simulink model "optimized_airport_sim_2"  (R2021a)
settings: Solver=VariableStepAuto  StartTime=0.0  StopTime=1e5  RelTol=1e-3
undefined symbols (not defined in the file): m, n
(part 1 of 2)
settings Model: Creator=hagarusama  LastModifiedBy=hagarusama

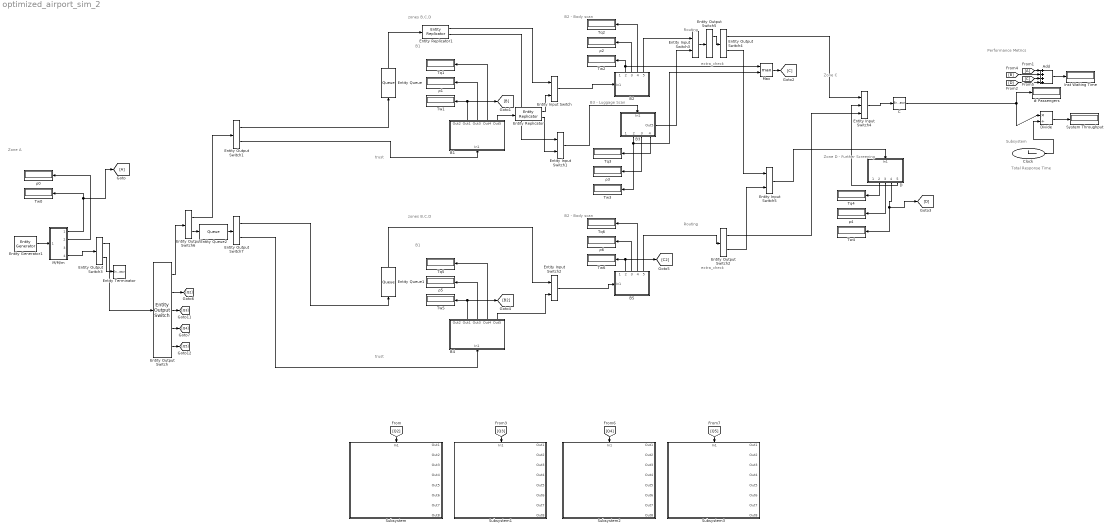
== system optimized_airport_sim_2 ==
  note: B1
  note: zones B,C,D
  note: Zone C
  note: B3 -
      | Luggage
      | Scan
  note: Subsystem
  note: Routing
  note: Zone D -
      |
      | Further
      | Screening
  note: Total Response Time
  note: B2 -
      | Body
      | scan
  note: Performance Metrics
  note: trust
  note: Zone A
  note: extra_check
  note: B1
  note: zones B,C,D
  note: Routing
  note: B2 -
      | Body
      | scan
  note: trust
  note: extra_check
  # Passengers : Display
  Add : Sum  Inputs=++++  SaturateOnIntegerOverflow=on
  B1 : Subsystem
  B2 : Subsystem
      settings: PortSchema="{\"entries\":[{\"content\":{\"sides\":[{\"content\":{\"connectorIds\":[]},\"type\":\"ConnectorPlacement.EquallySpacedRectSide\",\"uuid\":\"7ea955c4-59a0-4b16-a665-3c7419b36f79\"},{\"content\":{\"connectorIds\":[\"Out1\",\"Out2\",\"Out3\",\"Out4\",\"Out5\"],\"side\":\"RIGHT\"},\"type\":\"ConnectorPlacement.EquallySpacedRectSide\",\"uuid\":\"a8a3c229-e196-4360-bdfa-8ef645b2ce9c\"},{\"content\":{\"connectorIds\":[\"In1\"],\"side\":\"TOP\"},\"type\":\"ConnectorPlacement.EquallySpacedRectSide\",\"uuid\":\"5260f7b5-f6e8-463a-b0c5-598c56357d98\"}]},\"type\":\"ConnectorPlacement.EquallySpacedConnector\",\"uuid\":\"58c66fb9-1797-41d8-b8ed-62a065428871\"}],\"packageUris\":[\"http://schema.mathworks.com/mf0/Connector/R2020b\"],\"version\":\"1.0\"}"
  B3 : Subsystem
      settings: PortSchema="{\"entries\":[{\"content\":{\"sides\":[{\"content\":{\"connectorIds\":[\"In1\"]},\"type\":\"ConnectorPlacement.EquallySpacedRectSide\",\"uuid\":\"7ea955c4-59a0-4b16-a665-3c7419b36f79\"},{\"content\":{\"connectorIds\":[\"Out1\",\"Out2\",\"Out3\",\"Out4\"],\"side\":\"RIGHT\"},\"type\":\"ConnectorPlacement.EquallySpacedRectSide\",\"uuid\":\"a8a3c229-e196-4360-bdfa-8ef645b2ce9c\"},{\"content\":{\"connectorIds\":[],\"side\":\"TOP\"},\"type\":\"ConnectorPlacement.EquallySpacedRectSide\",\"uuid\":\"5260f7b5-f6e8-463a-b0c5-598c56357d98\"},{\"content\":{\"connectorIds\":[\"Out5\"],\"side\":\"BOTTOM\"},\"type\":\"ConnectorPlacement.EquallySpacedRectSide\",\"uuid\":\"b778f381-c9da-4203-8e39-7c353a561693\"}]},\"type\":\"ConnectorPlacement.EquallySpacedConnector\",\"uuid\":\"58c66fb9-1797-41d8-b8ed-62a065428871\"}],\"packageUris\":[\"http://schema.mathworks.com/mf0/Connector/R2020b\"],\"version\":\"1.0\"}"
  B4 : Subsystem
  B5 : Subsystem
      settings: PortSchema="{\"entries\":[{\"content\":{\"sides\":[{\"content\":{\"connectorIds\":[]},\"type\":\"ConnectorPlacement.EquallySpacedRectSide\",\"uuid\":\"7ea955c4-59a0-4b16-a665-3c7419b36f79\"},{\"content\":{\"connectorIds\":[\"Out1\",\"Out2\",\"Out3\",\"Out4\",\"Out5\"],\"side\":\"RIGHT\"},\"type\":\"ConnectorPlacement.EquallySpacedRectSide\",\"uuid\":\"a8a3c229-e196-4360-bdfa-8ef645b2ce9c\"},{\"content\":{\"connectorIds\":[\"In1\"],\"side\":\"TOP\"},\"type\":\"ConnectorPlacement.EquallySpacedRectSide\",\"uuid\":\"5260f7b5-f6e8-463a-b0c5-598c56357d98\"}]},\"type\":\"ConnectorPlacement.EquallySpacedConnector\",\"uuid\":\"58c66fb9-1797-41d8-b8ed-62a065428871\"}],\"packageUris\":[\"http://schema.mathworks.com/mf0/Connector/R2020b\"],\"version\":\"1.0\"}"
  C : EntityTerminator  InputPortMessageModes=m  NumberEntitiesArrived=on
      settings: OutputPortMap=o0
  Clock : Clock
  D : Subsystem
  Divide : Product  Inputs=*/  SaturateOnIntegerOverflow=on
  Entity Input Switch : EntityInputSwitch  InputPortMessageModes=m,m  OutputPortMessageModes=m
  Entity Input Switch1 : EntityInputSwitch  InputPortMessageModes=m,m  OutputPortMessageModes=m
  Entity Input Switch2 : EntityInputSwitch  InputPortMessageModes=m,m  OutputPortMessageModes=m
  Entity Input Switch3 : EntityInputSwitch  InputPortMessageModes=m,m  OutputPortMessageModes=m  ActivePortSelection=Switch  SwitchingCriterion=Equiprobable  Seed=450279
  Entity Input Switch4 : EntityInputSwitch  InputPortMessageModes=m,m,m  OutputPortMessageModes=m  NumberInputPorts=3  SwitchingCriterion=Equiprobable  Seed=450279
      settings: InputPortMap=u1,u2,u3
  Entity Input Switch5 : EntityInputSwitch  InputPortMessageModes=m,m  OutputPortMessageModes=m  SwitchingCriterion=Equiprobable  Seed=450279
  Entity Output Switch : EntityOutputSwitch  InputPortMessageModes=m  OutputPortMessageModes=m,m,m,m,m  NumberOutputPorts=5  SwitchingCriterion=Equiprobable  Seed=9647085  SwitchAttributeName=Attribute1
      settings: OutputPortMap=o0,o1,o2,o3,o4
  Entity Output Switch1 : EntityOutputSwitch  InputPortMessageModes=m  OutputPortMessageModes=m,m  SwitchingCriterion=From attribute  Seed=9647085  SwitchAttributeName=trust
  Entity Output Switch2 : EntityOutputSwitch  InputPortMessageModes=m  OutputPortMessageModes=m,m  SwitchingCriterion=From attribute  Seed=9632160  SwitchAttributeName=extra_check
  Entity Output Switch3 : EntityOutputSwitch  InputPortMessageModes=m  OutputPortMessageModes=m,m  SwitchingCriterion=From attribute  Seed=9647085  SwitchAttributeName=valid
  Entity Output Switch4 : EntityOutputSwitch  InputPortMessageModes=m  OutputPortMessageModes=m,m  SwitchingCriterion=From attribute  Seed=9632160  SwitchAttributeName=extra_check
  Entity Output Switch5 : EntityOutputSwitch  InputPortMessageModes=m  OutputPortMessageModes=m,m  SwitchingCriterion=Equiprobable  Seed=604377
  Entity Output Switch6 : EntityOutputSwitch  InputPortMessageModes=m  OutputPortMessageModes=m,m  SwitchingCriterion=From attribute  Seed=9647085  SwitchAttributeName=luggage
  Entity Output Switch7 : EntityOutputSwitch  InputPortMessageModes=m  OutputPortMessageModes=m,m  SwitchingCriterion=From attribute  Seed=9647085  SwitchAttributeName=trust
  Entity Generator1 : EntityGenerator  OutputPortMessageModes=m  TimeSource=MATLAB action  IntergenerationTimeAction=|  GenerateAction=|  AttributeName=trust|luggage|valid|extra_check|rand  AttributeInitialValue=1|1|1|1|0.9  EntityType=Structured  EntityTypeName=Entity
      IntergenerationTimeAction=|
      | dt = rand(1,1);
      | persistent rngInit;
      | if isempty(rngInit)
      |     seed = 153503;
      |     rng(seed);
      |     rngInit = true;
      | end
      | 
      | % Pattern: Exponential distribution
      | mu = 4;
      | dt = -mu * log(1 - rand());
      GenerateAction=|
      | % entity.trust = 2;
      | % entity.luggage = 1;
      | 
      | entity.rand = rand();
      |   if 0.02 <= entity.rand
      |      entity.extra_check = 1;
      |   else
      |      entity.extra_check = 2;
      |   end
      | 
      |   if 0.55 <= entity.rand
      |      entity.trust = 1;
      |   else
      |      entity.trust = 2;
      |   end
      | 
      |   if 0.2 <= entity.rand
      |      entity.luggage = 1;
      |   else
      |     entity.luggage = 2;
      |   end
  Entity Queue : Queue  InputPortMessageModes=m  OutputPortMessageModes=m  Capacity=inf
  Entity Queue1 : Queue  InputPortMessageModes=m  OutputPortMessageModes=m  Capacity=inf
  Entity Queue2 : Queue  InputPortMessageModes=m  OutputPortMessageModes=m  Capacity=Inf
  Entity Replicator : EntityReplicator  InputPortMessageModes=m  OutputPortMessageModes=m,m
  Entity Replicator1 : EntityReplicator  InputPortMessageModes=m  OutputPortMessageModes=m,m
  Entity Terminator : EntityTerminator  InputPortMessageModes=m
  Inst Waiting Time : Display
  M/M/m : Subsystem
  Max : MinMax  Function=max  Inputs=2
  Subsystem : Subsystem
      settings: PortSchema="{\"entries\":[{\"content\":{\"sides\":[{\"content\":{\"connectorIds\":[]},\"type\":\"ConnectorPlacement.EquallySpacedRectSide\",\"uuid\":\"1c08f6fe-4c87-411e-915d-6e2a500d8702\"},{\"content\":{\"connectorIds\":[\"Out1\",\"Out2\",\"Out3\",\"Out4\",\"Out5\",\"Out6\",\"Out7\",\"Out8\"],\"side\":\"RIGHT\"},\"type\":\"ConnectorPlacement.EquallySpacedRectSide\",\"uuid\":\"910b190e-7dcd-45fd-8ee8-821638941447\"},{\"content\":{\"connectorIds\":[\"In1\"],\"side\":\"TOP\"},\"type\":\"ConnectorPlacement.EquallySpacedRectSide\",\"uuid\":\"2ddee95e-0d30-4175-a05d-21c06b813b57\"}]},\"type\":\"ConnectorPlacement.EquallySpacedConnector\",\"uuid\":\"737bed06-a4bf-4b3a-b5a9-477a48340c42\"}],\"packageUris\":[\"http://schema.mathworks.com/mf0/Connector/R2020b\"],\"version\":\"1.0\"}"
  Subsystem1 : Subsystem
      settings: PortSchema="{\"entries\":[{\"content\":{\"sides\":[{\"content\":{\"connectorIds\":[]},\"type\":\"ConnectorPlacement.EquallySpacedRectSide\",\"uuid\":\"1c08f6fe-4c87-411e-915d-6e2a500d8702\"},{\"content\":{\"connectorIds\":[\"Out1\",\"Out2\",\"Out3\",\"Out4\",\"Out5\",\"Out6\",\"Out7\",\"Out8\"],\"side\":\"RIGHT\"},\"type\":\"ConnectorPlacement.EquallySpacedRectSide\",\"uuid\":\"910b190e-7dcd-45fd-8ee8-821638941447\"},{\"content\":{\"connectorIds\":[\"In1\"],\"side\":\"TOP\"},\"type\":\"ConnectorPlacement.EquallySpacedRectSide\",\"uuid\":\"2ddee95e-0d30-4175-a05d-21c06b813b57\"}]},\"type\":\"ConnectorPlacement.EquallySpacedConnector\",\"uuid\":\"737bed06-a4bf-4b3a-b5a9-477a48340c42\"}],\"packageUris\":[\"http://schema.mathworks.com/mf0/Connector/R2020b\"],\"version\":\"1.0\"}"
  Subsystem2 : Subsystem
      settings: PortSchema="{\"entries\":[{\"content\":{\"sides\":[{\"content\":{\"connectorIds\":[]},\"type\":\"ConnectorPlacement.EquallySpacedRectSide\",\"uuid\":\"1c08f6fe-4c87-411e-915d-6e2a500d8702\"},{\"content\":{\"connectorIds\":[\"Out1\",\"Out2\",\"Out3\",\"Out4\",\"Out5\",\"Out6\",\"Out7\",\"Out8\"],\"side\":\"RIGHT\"},\"type\":\"ConnectorPlacement.EquallySpacedRectSide\",\"uuid\":\"910b190e-7dcd-45fd-8ee8-821638941447\"},{\"content\":{\"connectorIds\":[\"In1\"],\"side\":\"TOP\"},\"type\":\"ConnectorPlacement.EquallySpacedRectSide\",\"uuid\":\"2ddee95e-0d30-4175-a05d-21c06b813b57\"}]},\"type\":\"ConnectorPlacement.EquallySpacedConnector\",\"uuid\":\"737bed06-a4bf-4b3a-b5a9-477a48340c42\"}],\"packageUris\":[\"http://schema.mathworks.com/mf0/Connector/R2020b\"],\"version\":\"1.0\"}"
  Subsystem3 : Subsystem
      settings: PortSchema="{\"entries\":[{\"content\":{\"sides\":[{\"content\":{\"connectorIds\":[]},\"type\":\"ConnectorPlacement.EquallySpacedRectSide\",\"uuid\":\"1c08f6fe-4c87-411e-915d-6e2a500d8702\"},{\"content\":{\"connectorIds\":[\"Out1\",\"Out2\",\"Out3\",\"Out4\",\"Out5\",\"Out6\",\"Out7\",\"Out8\"],\"side\":\"RIGHT\"},\"type\":\"ConnectorPlacement.EquallySpacedRectSide\",\"uuid\":\"910b190e-7dcd-45fd-8ee8-821638941447\"},{\"content\":{\"connectorIds\":[\"In1\"],\"side\":\"TOP\"},\"type\":\"ConnectorPlacement.EquallySpacedRectSide\",\"uuid\":\"2ddee95e-0d30-4175-a05d-21c06b813b57\"}]},\"type\":\"ConnectorPlacement.EquallySpacedConnector\",\"uuid\":\"737bed06-a4bf-4b3a-b5a9-477a48340c42\"}],\"packageUris\":[\"http://schema.mathworks.com/mf0/Connector/R2020b\"],\"version\":\"1.0\"}"
  System Throughput : Display
  Tq{1..6} (6 alike) : Display
  Tw{0..6} (7 alike) : Display
  ρ{0..6} (7 alike) : Display
  wires:
  B3/5(Out5) -> Entity Input Switch3/2
  [C] -> Add/3
  Entity Input Switch3/1 -> Entity Output Switch5/1
  B2/5(Out5) -> Entity Input Switch3/1
  Entity Queue/1 -> Entity Replicator1/1
  M/M/m/4(Out4) -> Entity Output Switch3/1
  B2/4(Out4) -> Tq2/1
  M/M/m/1(Out1) -> [A], Tw0/1
  Entity Output Switch5/1 -> Entity Output Switch4/1
  [A] -> Add/1
  Entity Replicator1/2 -> Entity Input Switch1/1
  Entity Output Switch3/1 -> Entity Output Switch/1
  M/M/m/2(Out2) -> ρ0/1
  Max/1 -> [C]
  Entity Output Switch3/2 -> Entity Terminator/1
  D/3(Out3) -> ρ4/1
  B1/4(Out4) -> Tq1/1
  B3/4(Out4) -> Tq3/1
  [D] -> Add/4
  Divide/1 -> System Throughput/1
  B2/2(Out1) -> Max/1, Tw2/1
  Entity Replicator1/1 -> Entity Input Switch/1
  Entity Output Switch1/1 -> Entity Queue/1
  Add/1 -> Inst Waiting Time/1
  B2/3(Out3) -> ρ2/1
  D/2(Out1) -> Tq4/1
  [B] -> Add/2
  B3/2(Out1) -> Tw3/1, Max/2
  B1/5(Out5) -> Entity Replicator/1
  Entity Generator1/1 -> M/M/m/1(In1)
  B1/3(Out3) -> ρ1/1
  Entity Output Switch4/1 -> Entity Input Switch4/1
  B1/2(Out1) -> Tw1/1, [B]
  Entity Input Switch/1 -> B2/1(In1)
  B3/3(Out3) -> ρ3/1
  Entity Replicator/2 -> Entity Input Switch1/2
  Clock/1 -> Divide/2
  Entity Output Switch1/2 -> B1/1(In1)
  Entity Replicator/1 -> Entity Input Switch/2
  D/4(Out4) -> Tw4/1, [D]
  Entity Output Switch/1 -> Entity Output Switch6/1
  Entity Output Switch6/1 -> Entity Output Switch1/1
  Entity Output Switch6/2 -> Entity Queue2/1
  Entity Queue2/1 -> Entity Output Switch7/1
  Entity Input Switch1/1 -> B3/1(In1)
  B4/5(Out5) -> Entity Input Switch2/2
  Entity Input Switch2/1 -> B5/1(In1)
  B4/2(Out1) -> [B2], Tw5/1
  B4/3(Out3) -> ρ5/1
  B5/3(Out3) -> ρ6/1
  Entity Output Switch7/1 -> Entity Queue1/1
  Entity Queue1/1 -> Entity Input Switch2/1
  B4/4(Out4) -> Tq5/1
  B5/2(Out1) -> [C2], Tw6/1
  B5/5(Out5) -> Entity Output Switch2/1
  B5/4(Out4) -> Tq6/1
  Entity Output Switch7/2 -> B4/1(In1)
  Entity Input Switch4/1 -> C/1
  D/5(Out5) -> Entity Input Switch4/2
  Entity Input Switch5/1 -> D/1(In1)
  Entity Output Switch4/2 -> Entity Input Switch5/1
  Entity Output Switch2/2 -> Entity Input Switch5/2
  C/1 -> Divide/1, # Passengers/1
  Entity Output Switch2/1 -> Entity Input Switch4/3
  Entity Output Switch/2 -> [Q2]
  Entity Output Switch/3 -> [Q3]
  [Q2] -> Subsystem/1(In1)
  [Q3] -> Subsystem1/1(In1)
  Entity Output Switch/5 -> [Q5]
  Entity Output Switch/4 -> [Q4]
  [Q5] -> Subsystem3/1(In1)
  [Q4] -> Subsystem2/1(In1)

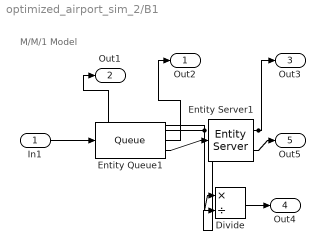
== system optimized_airport_sim_2/B1 ==
  note: M/M/1 Model
  In1 : Inport
  Divide : Product  Inputs=*/
  Entity Queue1 : Queue  InputPortMessageModes=m  OutputPortMessageModes=n,n,m  Capacity=inf  AverageWait=on  AverageQueueLength=on
      settings: OutputPortMap=o2,o3,o5
  Entity Server1 : EntityServer  InputPortMessageModes=m  OutputPortMessageModes=n,m  Capacity=1  ServiceTimeSource=MATLAB action  ServiceTimeAction=|  Utilization=on
      | dt = rand(1,1);
      | persistent rngInit;
      | if isempty(rngInit)
      |     seed = 2273520;
      |     rng(seed);
      |     rngInit = true;
      | end
      | 
      | % Pattern: Exponential distribution
      | mu = 15;
      | dt = -mu * log(1 - rand());
      settings: OutputPortMap=o5,o9
  Out2 : Outport
  Out1 : Outport  Port=2
  Out3 : Outport  Port=3
  Out4 : Outport  Port=4
  Out5 : Outport  Port=5
  wires:
  In1/1 -> Entity Queue1/1
  Entity Queue1/2 -> Out2/1
  Entity Server1/1 -> Divide/2, Out3/1
  Entity Queue1/1 -> Divide/1, Out1/1
  Entity Queue1/3 -> Entity Server1/1
  Entity Server1/2 -> Out5/1
  Divide/1 -> Out4/1

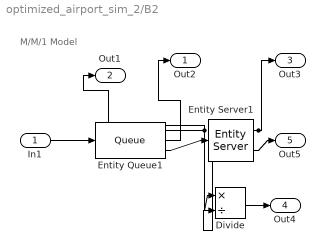
== system optimized_airport_sim_2/B2 ==
  note: M/M/1 Model
  In1 : Inport
  Divide : Product  Inputs=*/
  Entity Queue1 : Queue  InputPortMessageModes=m  OutputPortMessageModes=n,n,m  Capacity=inf  AverageWait=on  AverageQueueLength=on
      settings: OutputPortMap=o2,o3,o5
  Entity Server1 : EntityServer  InputPortMessageModes=m  OutputPortMessageModes=n,m  Capacity=1  ServiceTimeSource=MATLAB action  ServiceTimeAction=|  Utilization=on
      | dt = rand(1,1);
      | persistent rngInit;
      | if isempty(rngInit)
      |     seed = 7612432;
      |     rng(seed);
      |     rngInit = true;
      | end
      | 
      | % Pattern: Exponential distribution
      | mu = 5;
      | dt = -mu * log(1 - rand());
      settings: OutputPortMap=o5,o9
  Out2 : Outport
  Out1 : Outport  Port=2
  Out3 : Outport  Port=3
  Out4 : Outport  Port=4
  Out5 : Outport  Port=5
  wires:
  Divide/1 -> Out4/1
  Entity Server1/2 -> Out5/1
  Entity Queue1/3 -> Entity Server1/1
  Entity Queue1/1 -> Out1/1, Divide/1
  Entity Server1/1 -> Out3/1, Divide/2
  Entity Queue1/2 -> Out2/1
  In1/1 -> Entity Queue1/1

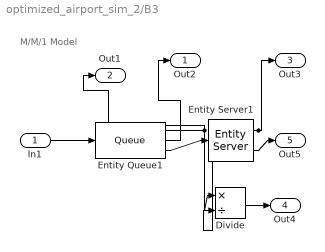
== system optimized_airport_sim_2/B3 ==
  note: M/M/1 Model
  In1 : Inport
  Divide : Product  Inputs=*/
  Entity Queue1 : Queue  InputPortMessageModes=m  OutputPortMessageModes=n,n,m  Capacity=inf  AverageWait=on  AverageQueueLength=on
      settings: OutputPortMap=o2,o3,o5
  Entity Server1 : EntityServer  InputPortMessageModes=m  OutputPortMessageModes=n,m  Capacity=1  ServiceTimeSource=MATLAB action  ServiceTimeAction=|  Utilization=on
      | dt = rand(1,1);
      | persistent rngInit;
      | if isempty(rngInit)
      |     seed = 6069205;
      |     rng(seed);
      |     rngInit = true;
      | end
      | 
      | % Pattern: Exponential distribution
      | mu = 8;
      | dt = -mu * log(1 - rand());
      settings: OutputPortMap=o5,o9
  Out2 : Outport
  Out1 : Outport  Port=2
  Out3 : Outport  Port=3
  Out4 : Outport  Port=4
  Out5 : Outport  Port=5
  wires:
  In1/1 -> Entity Queue1/1
  Entity Queue1/2 -> Out2/1
  Entity Server1/1 -> Divide/2, Out3/1
  Entity Queue1/1 -> Divide/1, Out1/1
  Entity Queue1/3 -> Entity Server1/1
  Entity Server1/2 -> Out5/1
  Divide/1 -> Out4/1

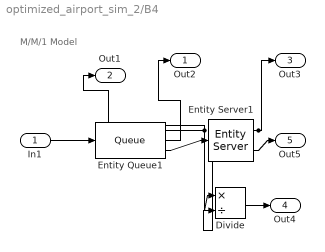
== system optimized_airport_sim_2/B4 ==
  note: M/M/1 Model
  In1 : Inport
  Divide : Product  Inputs=*/
  Entity Queue1 : Queue  InputPortMessageModes=m  OutputPortMessageModes=n,n,m  Capacity=inf  AverageWait=on  AverageQueueLength=on
      settings: OutputPortMap=o2,o3,o5
  Entity Server1 : EntityServer  InputPortMessageModes=m  OutputPortMessageModes=n,m  Capacity=1  ServiceTimeSource=MATLAB action  ServiceTimeAction=|  Utilization=on
      | dt = rand(1,1);
      | persistent rngInit;
      | if isempty(rngInit)
      |     seed = 2273520;
      |     rng(seed);
      |     rngInit = true;
      | end
      | 
      | % Pattern: Exponential distribution
      | mu = 10;
      | dt = -mu * log(1 - rand());
      settings: OutputPortMap=o5,o9
  Out2 : Outport
  Out1 : Outport  Port=2
  Out3 : Outport  Port=3
  Out4 : Outport  Port=4
  Out5 : Outport  Port=5
  wires:
  Divide/1 -> Out4/1
  Entity Server1/2 -> Out5/1
  Entity Queue1/3 -> Entity Server1/1
  Entity Queue1/1 -> Out1/1, Divide/1
  Entity Server1/1 -> Out3/1, Divide/2
  Entity Queue1/2 -> Out2/1
  In1/1 -> Entity Queue1/1

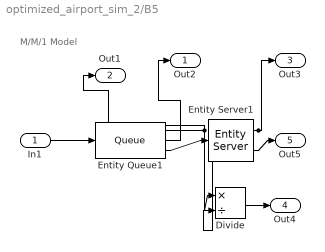
== system optimized_airport_sim_2/B5 ==
  note: M/M/1 Model
  In1 : Inport
  Divide : Product  Inputs=*/
  Entity Queue1 : Queue  InputPortMessageModes=m  OutputPortMessageModes=n,n,m  Capacity=inf  AverageWait=on  AverageQueueLength=on
      settings: OutputPortMap=o2,o3,o5
  Entity Server1 : EntityServer  InputPortMessageModes=m  OutputPortMessageModes=n,m  Capacity=1  ServiceTimeSource=MATLAB action  ServiceTimeAction=|  Utilization=on
      | dt = rand(1,1);
      | persistent rngInit;
      | if isempty(rngInit)
      |     seed = 7612432;
      |     rng(seed);
      |     rngInit = true;
      | end
      | 
      | % Pattern: Exponential distribution
      | mu = 5;
      | dt = -mu * log(1 - rand());
      settings: OutputPortMap=o5,o9
  Out2 : Outport
  Out1 : Outport  Port=2
  Out3 : Outport  Port=3
  Out4 : Outport  Port=4
  Out5 : Outport  Port=5
  wires:
  In1/1 -> Entity Queue1/1
  Entity Queue1/2 -> Out2/1
  Entity Server1/1 -> Divide/2, Out3/1
  Entity Queue1/1 -> Divide/1, Out1/1
  Entity Queue1/3 -> Entity Server1/1
  Entity Server1/2 -> Out5/1
  Divide/1 -> Out4/1

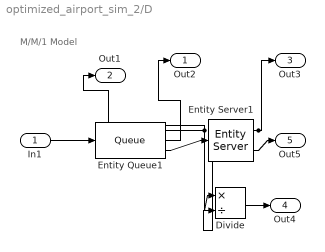
== system optimized_airport_sim_2/D ==
  note: M/M/1 Model
  In1 : Inport
  Divide : Product  Inputs=*/
  Entity Queue1 : Queue  InputPortMessageModes=m  OutputPortMessageModes=n,n,m  Capacity=inf  AverageWait=on  AverageQueueLength=on
      settings: OutputPortMap=o2,o3,o5
  Entity Server1 : EntityServer  InputPortMessageModes=m  OutputPortMessageModes=n,m  Capacity=1  ServiceTimeSource=MATLAB action  ServiceTimeAction=|  Utilization=on
      | dt = rand(1,1);
      | persistent rngInit;
      | if isempty(rngInit)
      |     seed = 6069205;
      |     rng(seed);
      |     rngInit = true;
      | end
      | 
      | % Pattern: Exponential distribution
      | mu = 60*3;
      | dt = -mu * log(1 - rand());
      settings: OutputPortMap=o5,o9
  Out2 : Outport
  Out1 : Outport  Port=2
  Out3 : Outport  Port=3
  Out4 : Outport  Port=4
  Out5 : Outport  Port=5
  wires:
  Divide/1 -> Out4/1
  Entity Server1/2 -> Out5/1
  Entity Queue1/3 -> Entity Server1/1
  Entity Queue1/1 -> Out1/1, Divide/1
  Entity Server1/1 -> Out3/1, Divide/2
  Entity Queue1/2 -> Out2/1
  In1/1 -> Entity Queue1/1

== system optimized_airport_sim_2/M//M//m ==
  note: M/M/m model
  In1 : Inport
  Entity Queue1 : Queue  InputPortMessageModes=m  OutputPortMessageModes=n,n,m  Capacity=inf  AverageWait=on  AverageQueueLength=on
      settings: OutputPortMap=o2,o3,o5
  Entity Server1 : EntityServer  InputPortMessageModes=m  OutputPortMessageModes=n,m  ServiceTimeSource=MATLAB action  ServiceTimeAction=|  ServiceCompleteAction=|  Utilization=on
      ServiceTimeAction=|
      | dt = rand(1,1);
      | persistent rngInit;
      | if isempty(rngInit)
      |     seed = 8084213;
      |     rng(seed);
      |     rngInit = true;
      | end
      | 
      | % Pattern: Exponential distribution
      | mu = 10;
      | dt = -mu * log(1 - rand());
      ServiceCompleteAction=|
      | if 0.15 <= rand()
      |   entity.valid = 1;
      | else
      |   entity.valid =2;
      | end
      settings: OutputPortMap=o5,o9
  Out1 : Outport
  Out2 : Outport  Port=2
  Out3 : Outport  Port=3
  Out4 : Outport  Port=4
  wires:
  Entity Queue1/3 -> Entity Server1/1
  Entity Queue1/1 -> Out3/1
  In1/1 -> Entity Queue1/1
  Entity Queue1/2 -> Out1/1
  Entity Server1/2 -> Out4/1
  Entity Server1/1 -> Out2/1

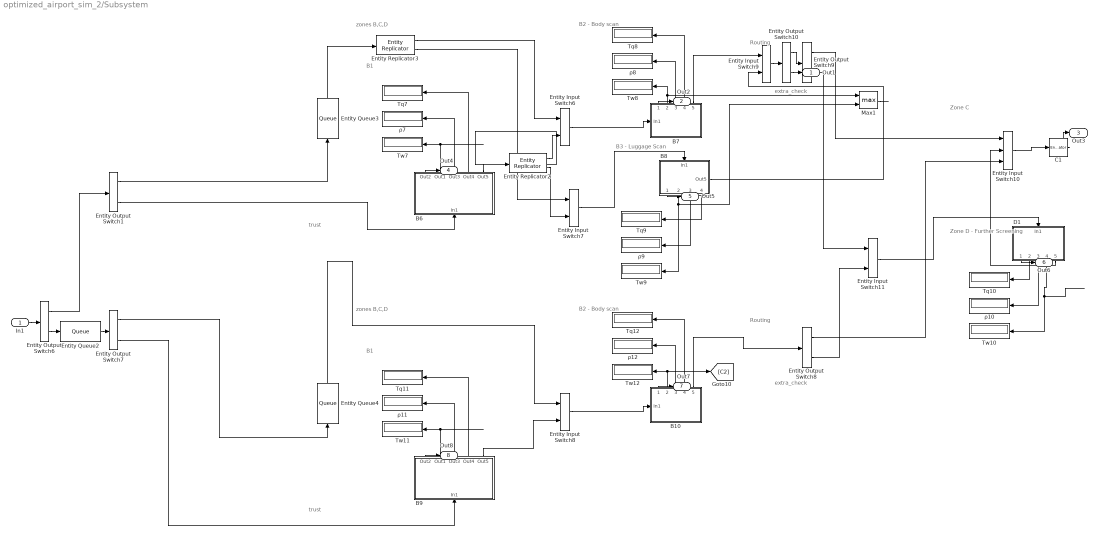
== system optimized_airport_sim_2/Subsystem ==
  note: B1
  note: zones B,C,D
  note: Zone C
  note: B3 -
      | Luggage
      | Scan
  note: Routing
  note: Zone D -
      |
      | Further
      | Screening
  note: B2 -
      | Body
      | scan
  note: trust
  note: extra_check
  note: B1
  note: zones B,C,D
  note: Routing
  note: B2 -
      | Body
      | scan
  note: trust
  note: extra_check
  In1 : Inport
  B10 : Subsystem
      settings: PortSchema="{\"entries\":[{\"content\":{\"sides\":[{\"content\":{\"connectorIds\":[]},\"type\":\"ConnectorPlacement.EquallySpacedRectSide\",\"uuid\":\"7ea955c4-59a0-4b16-a665-3c7419b36f79\"},{\"content\":{\"connectorIds\":[\"Out1\",\"Out2\",\"Out3\",\"Out4\",\"Out5\"],\"side\":\"RIGHT\"},\"type\":\"ConnectorPlacement.EquallySpacedRectSide\",\"uuid\":\"a8a3c229-e196-4360-bdfa-8ef645b2ce9c\"},{\"content\":{\"connectorIds\":[\"In1\"],\"side\":\"TOP\"},\"type\":\"ConnectorPlacement.EquallySpacedRectSide\",\"uuid\":\"5260f7b5-f6e8-463a-b0c5-598c56357d98\"}]},\"type\":\"ConnectorPlacement.EquallySpacedConnector\",\"uuid\":\"58c66fb9-1797-41d8-b8ed-62a065428871\"}],\"packageUris\":[\"http://schema.mathworks.com/mf0/Connector/R2020b\"],\"version\":\"1.0\"}"
  B6 : Subsystem
  B7 : Subsystem
      settings: PortSchema="{\"entries\":[{\"content\":{\"sides\":[{\"content\":{\"connectorIds\":[]},\"type\":\"ConnectorPlacement.EquallySpacedRectSide\",\"uuid\":\"7ea955c4-59a0-4b16-a665-3c7419b36f79\"},{\"content\":{\"connectorIds\":[\"Out1\",\"Out2\",\"Out3\",\"Out4\",\"Out5\"],\"side\":\"RIGHT\"},\"type\":\"ConnectorPlacement.EquallySpacedRectSide\",\"uuid\":\"a8a3c229-e196-4360-bdfa-8ef645b2ce9c\"},{\"content\":{\"connectorIds\":[\"In1\"],\"side\":\"TOP\"},\"type\":\"ConnectorPlacement.EquallySpacedRectSide\",\"uuid\":\"5260f7b5-f6e8-463a-b0c5-598c56357d98\"}]},\"type\":\"ConnectorPlacement.EquallySpacedConnector\",\"uuid\":\"58c66fb9-1797-41d8-b8ed-62a065428871\"}],\"packageUris\":[\"http://schema.mathworks.com/mf0/Connector/R2020b\"],\"version\":\"1.0\"}"
  B8 : Subsystem
      settings: PortSchema="{\"entries\":[{\"content\":{\"sides\":[{\"content\":{\"connectorIds\":[\"In1\"]},\"type\":\"ConnectorPlacement.EquallySpacedRectSide\",\"uuid\":\"7ea955c4-59a0-4b16-a665-3c7419b36f79\"},{\"content\":{\"connectorIds\":[\"Out1\",\"Out2\",\"Out3\",\"Out4\"],\"side\":\"RIGHT\"},\"type\":\"ConnectorPlacement.EquallySpacedRectSide\",\"uuid\":\"a8a3c229-e196-4360-bdfa-8ef645b2ce9c\"},{\"content\":{\"connectorIds\":[],\"side\":\"TOP\"},\"type\":\"ConnectorPlacement.EquallySpacedRectSide\",\"uuid\":\"5260f7b5-f6e8-463a-b0c5-598c56357d98\"},{\"content\":{\"connectorIds\":[\"Out5\"],\"side\":\"BOTTOM\"},\"type\":\"ConnectorPlacement.EquallySpacedRectSide\",\"uuid\":\"b778f381-c9da-4203-8e39-7c353a561693\"}]},\"type\":\"ConnectorPlacement.EquallySpacedConnector\",\"uuid\":\"58c66fb9-1797-41d8-b8ed-62a065428871\"}],\"packageUris\":[\"http://schema.mathworks.com/mf0/Connector/R2020b\"],\"version\":\"1.0\"}"
  B9 : Subsystem
  C1 : EntityTerminator  InputPortMessageModes=m  NumberEntitiesArrived=on
      settings: OutputPortMap=o0
  D1 : Subsystem
  Entity Input Switch10 : EntityInputSwitch  InputPortMessageModes=m,m,m  OutputPortMessageModes=m  NumberInputPorts=3  SwitchingCriterion=Equiprobable  Seed=450279
      settings: InputPortMap=u1,u2,u3
  Entity Input Switch11 : EntityInputSwitch  InputPortMessageModes=m,m  OutputPortMessageModes=m  SwitchingCriterion=Equiprobable  Seed=450279
  Entity Input Switch6 : EntityInputSwitch  InputPortMessageModes=m,m  OutputPortMessageModes=m
  Entity Input Switch7 : EntityInputSwitch  InputPortMessageModes=m,m  OutputPortMessageModes=m
  Entity Input Switch8 : EntityInputSwitch  InputPortMessageModes=m,m  OutputPortMessageModes=m
  Entity Input Switch9 : EntityInputSwitch  InputPortMessageModes=m,m  OutputPortMessageModes=m  ActivePortSelection=Switch  SwitchingCriterion=Equiprobable  Seed=450279
  Entity Output Switch1 : EntityOutputSwitch  InputPortMessageModes=m  OutputPortMessageModes=m,m  SwitchingCriterion=From attribute  Seed=9647085  SwitchAttributeName=trust
  Entity Output Switch10 : EntityOutputSwitch  InputPortMessageModes=m  OutputPortMessageModes=m,m  SwitchingCriterion=Equiprobable  Seed=604377
  Entity Output Switch6 : EntityOutputSwitch  InputPortMessageModes=m  OutputPortMessageModes=m,m  SwitchingCriterion=From attribute  Seed=9647085  SwitchAttributeName=luggage
  Entity Output Switch7 : EntityOutputSwitch  InputPortMessageModes=m  OutputPortMessageModes=m,m  SwitchingCriterion=From attribute  Seed=9647085  SwitchAttributeName=trust
  Entity Output Switch8 : EntityOutputSwitch  InputPortMessageModes=m  OutputPortMessageModes=m,m  SwitchingCriterion=From attribute  Seed=9632160  SwitchAttributeName=extra_check
  Entity Output Switch9 : EntityOutputSwitch  InputPortMessageModes=m  OutputPortMessageModes=m,m  SwitchingCriterion=From attribute  Seed=9632160  SwitchAttributeName=extra_check
  Entity Queue2 : Queue  InputPortMessageModes=m  OutputPortMessageModes=m  Capacity=Inf
  Entity Queue3 : Queue  InputPortMessageModes=m  OutputPortMessageModes=m  Capacity=inf
  Entity Queue4 : Queue  InputPortMessageModes=m  OutputPortMessageModes=m  Capacity=inf
  Entity Replicator2 : EntityReplicator  InputPortMessageModes=m  OutputPortMessageModes=m,m
  Entity Replicator3 : EntityReplicator  InputPortMessageModes=m  OutputPortMessageModes=m,m
  Max1 : MinMax  Function=max  Inputs=2
  Tq{7..12} (6 alike) : Display
  Tw{7..12} (6 alike) : Display
  ρ{7..12} (6 alike) : Display
  Out1 : Outport
  Out2 : Outport  Port=2
  Out3 : Outport  Port=3
  Out4 : Outport  Port=4
  Out5 : Outport  Port=5
  Out6 : Outport  Port=6
  Out7 : Outport  Port=7
  Out8 : Outport  Port=8
  wires:
  B10/4(Out4) -> Tq12/1
  B8/3(Out3) -> ρ9/1
  Entity Output Switch8/1 -> Entity Input Switch10/3
  C1/1 -> Out3/1
  Entity Output Switch1/2 -> B6/1(In1)
  Entity Input Switch10/1 -> C1/1
  B7/2(Out1) -> Tw8/1, Max1/1
  B10/5(Out5) -> Entity Output Switch8/1
  Max1/1 -> ?
  Entity Input Switch9/1 -> Entity Output Switch10/1
  Entity Output Switch9/2 -> Entity Input Switch11/1
  D1/5(Out5) -> Entity Input Switch10/2
  B8/5(Out5) -> Entity Input Switch9/2
  Entity Input Switch11/1 -> D1/1(In1)
  B9/2(Out1) -> Tw11/1
  Entity Output Switch8/2 -> Entity Input Switch11/2
  B10/3(Out3) -> ρ12/1
  B6/5(Out5) -> Entity Replicator2/1
  B10/2(Out1) -> Tw12/1, [C2]
  Entity Input Switch8/1 -> B10/1(In1)
  B9/4(Out4) -> Tq11/1
  Entity Replicator3/2 -> Entity Input Switch7/1
  D1/1(Out2) -> Out6/1
  B6/2(Out1) -> Tw7/1
  B9/3(Out3) -> ρ11/1
  B9/5(Out5) -> Entity Input Switch8/2
  Entity Queue4/1 -> Entity Input Switch8/1
  B6/1(Out2) -> Out4/1
  D1/3(Out3) -> ρ10/1
  Entity Input Switch7/1 -> B8/1(In1)
  Entity Replicator2/2 -> Entity Input Switch7/2
  D1/4(Out4) -> Tw10/1
  Entity Replicator2/1 -> Entity Input Switch6/2
  Entity Queue3/1 -> Entity Replicator3/1
  Entity Input Switch6/1 -> B7/1(In1)
  B8/1(Out2) -> Out5/1
  B8/2(Out1) -> Max1/2, Tw9/1
  Entity Replicator3/1 -> Entity Input Switch6/1
  B7/3(Out3) -> ρ8/1
  D1/2(Out1) -> Tq10/1
  B9/1(Out2) -> Out8/1
  B6/3(Out3) -> ρ7/1
  Entity Output Switch9/1 -> Entity Input Switch10/1
  B10/1(Out2) -> Out7/1
  B8/4(Out4) -> Tq9/1
  B7/5(Out5) -> Entity Input Switch9/1
  B6/4(Out4) -> Tq7/1
  Entity Output Switch10/1 -> Entity Output Switch9/1
  B7/4(Out4) -> Tq8/1
  Entity Output Switch10/2 -> Out1/1
  B7/1(Out2) -> Out2/1
  Entity Output Switch1/1 -> Entity Queue3/1
  Entity Output Switch7/1 -> Entity Queue4/1
  Entity Output Switch6/2 -> Entity Queue2/1
  Entity Output Switch6/1 -> Entity Output Switch1/1
  Entity Output Switch7/2 -> B9/1(In1)
  Entity Queue2/1 -> Entity Output Switch7/1
  In1/1 -> Entity Output Switch6/1

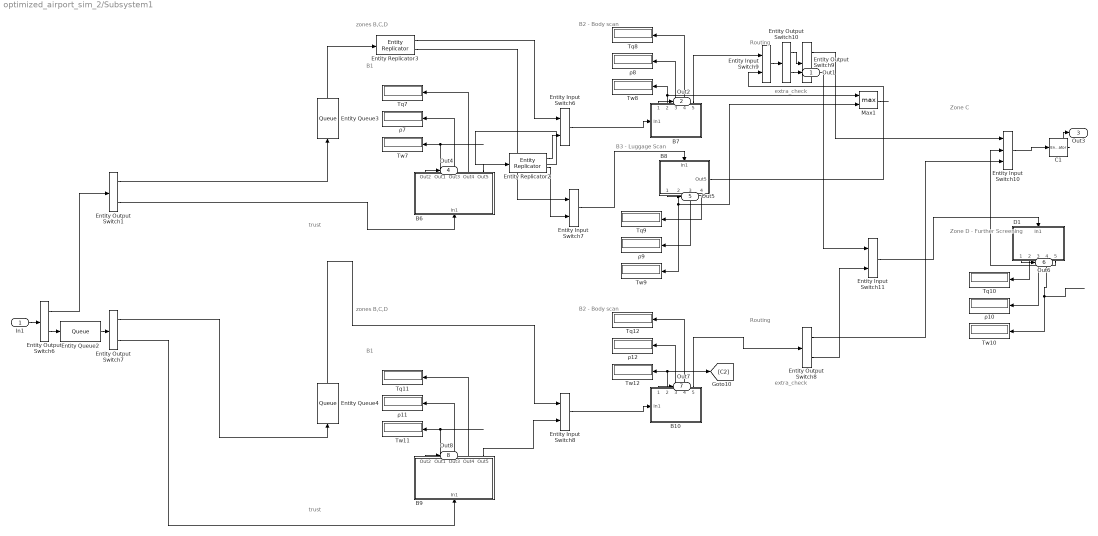
== system optimized_airport_sim_2/Subsystem1 ==
  note: extra_check
  note: trust
  note: B2 -
      | Body
      | scan
  note: Routing
  note: zones B,C,D
  note: B1
  note: extra_check
  note: trust
  note: B2 -
      | Body
      | scan
  note: Zone D -
      |
      | Further
      | Screening
  note: Routing
  note: B3 -
      | Luggage
      | Scan
  note: Zone C
  note: zones B,C,D
  note: B1
  In1 : Inport
  B10 : Subsystem
      settings: PortSchema="{\"entries\":[{\"content\":{\"sides\":[{\"content\":{\"connectorIds\":[]},\"type\":\"ConnectorPlacement.EquallySpacedRectSide\",\"uuid\":\"7ea955c4-59a0-4b16-a665-3c7419b36f79\"},{\"content\":{\"connectorIds\":[\"Out1\",\"Out2\",\"Out3\",\"Out4\",\"Out5\"],\"side\":\"RIGHT\"},\"type\":\"ConnectorPlacement.EquallySpacedRectSide\",\"uuid\":\"a8a3c229-e196-4360-bdfa-8ef645b2ce9c\"},{\"content\":{\"connectorIds\":[\"In1\"],\"side\":\"TOP\"},\"type\":\"ConnectorPlacement.EquallySpacedRectSide\",\"uuid\":\"5260f7b5-f6e8-463a-b0c5-598c56357d98\"}]},\"type\":\"ConnectorPlacement.EquallySpacedConnector\",\"uuid\":\"58c66fb9-1797-41d8-b8ed-62a065428871\"}],\"packageUris\":[\"http://schema.mathworks.com/mf0/Connector/R2020b\"],\"version\":\"1.0\"}"
  B6 : Subsystem
  B7 : Subsystem
      settings: PortSchema="{\"entries\":[{\"content\":{\"sides\":[{\"content\":{\"connectorIds\":[]},\"type\":\"ConnectorPlacement.EquallySpacedRectSide\",\"uuid\":\"7ea955c4-59a0-4b16-a665-3c7419b36f79\"},{\"content\":{\"connectorIds\":[\"Out1\",\"Out2\",\"Out3\",\"Out4\",\"Out5\"],\"side\":\"RIGHT\"},\"type\":\"ConnectorPlacement.EquallySpacedRectSide\",\"uuid\":\"a8a3c229-e196-4360-bdfa-8ef645b2ce9c\"},{\"content\":{\"connectorIds\":[\"In1\"],\"side\":\"TOP\"},\"type\":\"ConnectorPlacement.EquallySpacedRectSide\",\"uuid\":\"5260f7b5-f6e8-463a-b0c5-598c56357d98\"}]},\"type\":\"ConnectorPlacement.EquallySpacedConnector\",\"uuid\":\"58c66fb9-1797-41d8-b8ed-62a065428871\"}],\"packageUris\":[\"http://schema.mathworks.com/mf0/Connector/R2020b\"],\"version\":\"1.0\"}"
  B8 : Subsystem
      settings: PortSchema="{\"entries\":[{\"content\":{\"sides\":[{\"content\":{\"connectorIds\":[\"In1\"]},\"type\":\"ConnectorPlacement.EquallySpacedRectSide\",\"uuid\":\"7ea955c4-59a0-4b16-a665-3c7419b36f79\"},{\"content\":{\"connectorIds\":[\"Out1\",\"Out2\",\"Out3\",\"Out4\"],\"side\":\"RIGHT\"},\"type\":\"ConnectorPlacement.EquallySpacedRectSide\",\"uuid\":\"a8a3c229-e196-4360-bdfa-8ef645b2ce9c\"},{\"content\":{\"connectorIds\":[],\"side\":\"TOP\"},\"type\":\"ConnectorPlacement.EquallySpacedRectSide\",\"uuid\":\"5260f7b5-f6e8-463a-b0c5-598c56357d98\"},{\"content\":{\"connectorIds\":[\"Out5\"],\"side\":\"BOTTOM\"},\"type\":\"ConnectorPlacement.EquallySpacedRectSide\",\"uuid\":\"b778f381-c9da-4203-8e39-7c353a561693\"}]},\"type\":\"ConnectorPlacement.EquallySpacedConnector\",\"uuid\":\"58c66fb9-1797-41d8-b8ed-62a065428871\"}],\"packageUris\":[\"http://schema.mathworks.com/mf0/Connector/R2020b\"],\"version\":\"1.0\"}"
  B9 : Subsystem
  C1 : EntityTerminator  InputPortMessageModes=m  NumberEntitiesArrived=on
      settings: OutputPortMap=o0
  D1 : Subsystem
  Entity Input Switch10 : EntityInputSwitch  InputPortMessageModes=m,m,m  OutputPortMessageModes=m  NumberInputPorts=3  SwitchingCriterion=Equiprobable  Seed=450279
      settings: InputPortMap=u1,u2,u3
  Entity Input Switch11 : EntityInputSwitch  InputPortMessageModes=m,m  OutputPortMessageModes=m  SwitchingCriterion=Equiprobable  Seed=450279
  Entity Input Switch6 : EntityInputSwitch  InputPortMessageModes=m,m  OutputPortMessageModes=m
  Entity Input Switch7 : EntityInputSwitch  InputPortMessageModes=m,m  OutputPortMessageModes=m
  Entity Input Switch8 : EntityInputSwitch  InputPortMessageModes=m,m  OutputPortMessageModes=m
  Entity Input Switch9 : EntityInputSwitch  InputPortMessageModes=m,m  OutputPortMessageModes=m  ActivePortSelection=Switch  SwitchingCriterion=Equiprobable  Seed=450279
  Entity Output Switch1 : EntityOutputSwitch  InputPortMessageModes=m  OutputPortMessageModes=m,m  SwitchingCriterion=From attribute  Seed=9647085  SwitchAttributeName=trust
  Entity Output Switch10 : EntityOutputSwitch  InputPortMessageModes=m  OutputPortMessageModes=m,m  SwitchingCriterion=Equiprobable  Seed=604377
  Entity Output Switch6 : EntityOutputSwitch  InputPortMessageModes=m  OutputPortMessageModes=m,m  SwitchingCriterion=From attribute  Seed=9647085  SwitchAttributeName=luggage
  Entity Output Switch7 : EntityOutputSwitch  InputPortMessageModes=m  OutputPortMessageModes=m,m  SwitchingCriterion=From attribute  Seed=9647085  SwitchAttributeName=trust
  Entity Output Switch8 : EntityOutputSwitch  InputPortMessageModes=m  OutputPortMessageModes=m,m  SwitchingCriterion=From attribute  Seed=9632160  SwitchAttributeName=extra_check
  Entity Output Switch9 : EntityOutputSwitch  InputPortMessageModes=m  OutputPortMessageModes=m,m  SwitchingCriterion=From attribute  Seed=9632160  SwitchAttributeName=extra_check
  Entity Queue2 : Queue  InputPortMessageModes=m  OutputPortMessageModes=m  Capacity=Inf
  Entity Queue3 : Queue  InputPortMessageModes=m  OutputPortMessageModes=m  Capacity=inf
  Entity Queue4 : Queue  InputPortMessageModes=m  OutputPortMessageModes=m  Capacity=inf
  Entity Replicator2 : EntityReplicator  InputPortMessageModes=m  OutputPortMessageModes=m,m
  Entity Replicator3 : EntityReplicator  InputPortMessageModes=m  OutputPortMessageModes=m,m
  Max1 : MinMax  Function=max  Inputs=2
  Tq{7..12} (6 alike) : Display
  Tw{7..12} (6 alike) : Display
  ρ{7..12} (6 alike) : Display
  Out1 : Outport
  Out2 : Outport  Port=2
  Out3 : Outport  Port=3
  Out4 : Outport  Port=4
  Out5 : Outport  Port=5
  Out6 : Outport  Port=6
  Out7 : Outport  Port=7
  Out8 : Outport  Port=8
  wires:
  In1/1 -> Entity Output Switch6/1
  Entity Queue2/1 -> Entity Output Switch7/1
  Entity Output Switch7/2 -> B9/1(In1)
  Entity Output Switch6/1 -> Entity Output Switch1/1
  Entity Output Switch6/2 -> Entity Queue2/1
  Entity Output Switch7/1 -> Entity Queue4/1
  Entity Output Switch1/1 -> Entity Queue3/1
  B7/1(Out2) -> Out2/1
  Entity Output Switch10/2 -> Out1/1
  B7/4(Out4) -> Tq8/1
  Entity Output Switch10/1 -> Entity Output Switch9/1
  B6/4(Out4) -> Tq7/1
  B7/5(Out5) -> Entity Input Switch9/1
  B8/4(Out4) -> Tq9/1
  B10/1(Out2) -> Out7/1
  Entity Output Switch9/1 -> Entity Input Switch10/1
  B6/3(Out3) -> ρ7/1
  B9/1(Out2) -> Out8/1
  D1/2(Out1) -> Tq10/1
  B7/3(Out3) -> ρ8/1
  Entity Replicator3/1 -> Entity Input Switch6/1
  B8/2(Out1) -> Tw9/1, Max1/2
  B8/1(Out2) -> Out5/1
  Entity Input Switch6/1 -> B7/1(In1)
  Entity Queue3/1 -> Entity Replicator3/1
  Entity Replicator2/1 -> Entity Input Switch6/2
  D1/4(Out4) -> Tw10/1
  Entity Replicator2/2 -> Entity Input Switch7/2
  Entity Input Switch7/1 -> B8/1(In1)
  D1/3(Out3) -> ρ10/1
  B6/1(Out2) -> Out4/1
  Entity Queue4/1 -> Entity Input Switch8/1
  B9/5(Out5) -> Entity Input Switch8/2
  B9/3(Out3) -> ρ11/1
  B6/2(Out1) -> Tw7/1
  D1/1(Out2) -> Out6/1
  Entity Replicator3/2 -> Entity Input Switch7/1
  B9/4(Out4) -> Tq11/1
  Entity Input Switch8/1 -> B10/1(In1)
  B10/2(Out1) -> [C2], Tw12/1
  B6/5(Out5) -> Entity Replicator2/1
  B10/3(Out3) -> ρ12/1
  Entity Output Switch8/2 -> Entity Input Switch11/2
  B9/2(Out1) -> Tw11/1
  Entity Input Switch11/1 -> D1/1(In1)
  B8/5(Out5) -> Entity Input Switch9/2
  D1/5(Out5) -> Entity Input Switch10/2
  Entity Output Switch9/2 -> Entity Input Switch11/1
  Entity Input Switch9/1 -> Entity Output Switch10/1
  Max1/1 -> ?
  B10/5(Out5) -> Entity Output Switch8/1
  B7/2(Out1) -> Max1/1, Tw8/1
  Entity Input Switch10/1 -> C1/1
  Entity Output Switch1/2 -> B6/1(In1)
  C1/1 -> Out3/1
  Entity Output Switch8/1 -> Entity Input Switch10/3
  B8/3(Out3) -> ρ9/1
  B10/4(Out4) -> Tq12/1

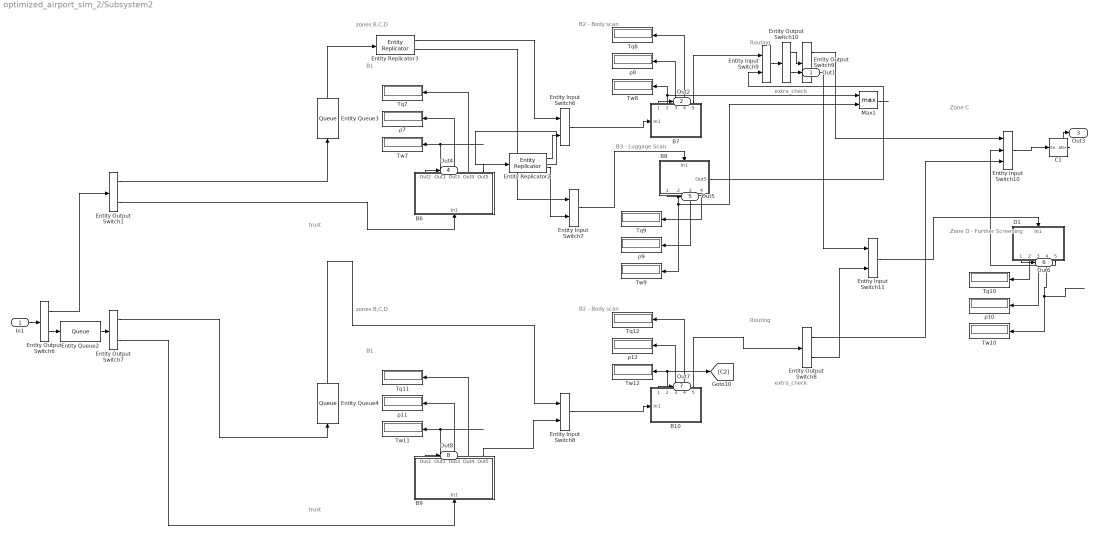
== system optimized_airport_sim_2/Subsystem2 ==
  note: extra_check
  note: trust
  note: B2 -
      | Body
      | scan
  note: Routing
  note: zones B,C,D
  note: B1
  note: extra_check
  note: trust
  note: B2 -
      | Body
      | scan
  note: Zone D -
      |
      | Further
      | Screening
  note: Routing
  note: B3 -
      | Luggage
      | Scan
  note: Zone C
  note: zones B,C,D
  note: B1
  In1 : Inport
  B10 : Subsystem
      settings: PortSchema="{\"entries\":[{\"content\":{\"sides\":[{\"content\":{\"connectorIds\":[]},\"type\":\"ConnectorPlacement.EquallySpacedRectSide\",\"uuid\":\"7ea955c4-59a0-4b16-a665-3c7419b36f79\"},{\"content\":{\"connectorIds\":[\"Out1\",\"Out2\",\"Out3\",\"Out4\",\"Out5\"],\"side\":\"RIGHT\"},\"type\":\"ConnectorPlacement.EquallySpacedRectSide\",\"uuid\":\"a8a3c229-e196-4360-bdfa-8ef645b2ce9c\"},{\"content\":{\"connectorIds\":[\"In1\"],\"side\":\"TOP\"},\"type\":\"ConnectorPlacement.EquallySpacedRectSide\",\"uuid\":\"5260f7b5-f6e8-463a-b0c5-598c56357d98\"}]},\"type\":\"ConnectorPlacement.EquallySpacedConnector\",\"uuid\":\"58c66fb9-1797-41d8-b8ed-62a065428871\"}],\"packageUris\":[\"http://schema.mathworks.com/mf0/Connector/R2020b\"],\"version\":\"1.0\"}"
  B6 : Subsystem
  B7 : Subsystem
      settings: PortSchema="{\"entries\":[{\"content\":{\"sides\":[{\"content\":{\"connectorIds\":[]},\"type\":\"ConnectorPlacement.EquallySpacedRectSide\",\"uuid\":\"7ea955c4-59a0-4b16-a665-3c7419b36f79\"},{\"content\":{\"connectorIds\":[\"Out1\",\"Out2\",\"Out3\",\"Out4\",\"Out5\"],\"side\":\"RIGHT\"},\"type\":\"ConnectorPlacement.EquallySpacedRectSide\",\"uuid\":\"a8a3c229-e196-4360-bdfa-8ef645b2ce9c\"},{\"content\":{\"connectorIds\":[\"In1\"],\"side\":\"TOP\"},\"type\":\"ConnectorPlacement.EquallySpacedRectSide\",\"uuid\":\"5260f7b5-f6e8-463a-b0c5-598c56357d98\"}]},\"type\":\"ConnectorPlacement.EquallySpacedConnector\",\"uuid\":\"58c66fb9-1797-41d8-b8ed-62a065428871\"}],\"packageUris\":[\"http://schema.mathworks.com/mf0/Connector/R2020b\"],\"version\":\"1.0\"}"
  B8 : Subsystem
      settings: PortSchema="{\"entries\":[{\"content\":{\"sides\":[{\"content\":{\"connectorIds\":[\"In1\"]},\"type\":\"ConnectorPlacement.EquallySpacedRectSide\",\"uuid\":\"7ea955c4-59a0-4b16-a665-3c7419b36f79\"},{\"content\":{\"connectorIds\":[\"Out1\",\"Out2\",\"Out3\",\"Out4\"],\"side\":\"RIGHT\"},\"type\":\"ConnectorPlacement.EquallySpacedRectSide\",\"uuid\":\"a8a3c229-e196-4360-bdfa-8ef645b2ce9c\"},{\"content\":{\"connectorIds\":[],\"side\":\"TOP\"},\"type\":\"ConnectorPlacement.EquallySpacedRectSide\",\"uuid\":\"5260f7b5-f6e8-463a-b0c5-598c56357d98\"},{\"content\":{\"connectorIds\":[\"Out5\"],\"side\":\"BOTTOM\"},\"type\":\"ConnectorPlacement.EquallySpacedRectSide\",\"uuid\":\"b778f381-c9da-4203-8e39-7c353a561693\"}]},\"type\":\"ConnectorPlacement.EquallySpacedConnector\",\"uuid\":\"58c66fb9-1797-41d8-b8ed-62a065428871\"}],\"packageUris\":[\"http://schema.mathworks.com/mf0/Connector/R2020b\"],\"version\":\"1.0\"}"
  B9 : Subsystem
  C1 : EntityTerminator  InputPortMessageModes=m  NumberEntitiesArrived=on
      settings: OutputPortMap=o0
  D1 : Subsystem
  Entity Input Switch10 : EntityInputSwitch  InputPortMessageModes=m,m,m  OutputPortMessageModes=m  NumberInputPorts=3  SwitchingCriterion=Equiprobable  Seed=450279
      settings: InputPortMap=u1,u2,u3
  Entity Input Switch11 : EntityInputSwitch  InputPortMessageModes=m,m  OutputPortMessageModes=m  SwitchingCriterion=Equiprobable  Seed=450279
  Entity Input Switch6 : EntityInputSwitch  InputPortMessageModes=m,m  OutputPortMessageModes=m
  Entity Input Switch7 : EntityInputSwitch  InputPortMessageModes=m,m  OutputPortMessageModes=m
  Entity Input Switch8 : EntityInputSwitch  InputPortMessageModes=m,m  OutputPortMessageModes=m
  Entity Input Switch9 : EntityInputSwitch  InputPortMessageModes=m,m  OutputPortMessageModes=m  ActivePortSelection=Switch  SwitchingCriterion=Equiprobable  Seed=450279
  Entity Output Switch1 : EntityOutputSwitch  InputPortMessageModes=m  OutputPortMessageModes=m,m  SwitchingCriterion=From attribute  Seed=9647085  SwitchAttributeName=trust
  Entity Output Switch10 : EntityOutputSwitch  InputPortMessageModes=m  OutputPortMessageModes=m,m  SwitchingCriterion=Equiprobable  Seed=604377
  Entity Output Switch6 : EntityOutputSwitch  InputPortMessageModes=m  OutputPortMessageModes=m,m  SwitchingCriterion=From attribute  Seed=9647085  SwitchAttributeName=luggage
  Entity Output Switch7 : EntityOutputSwitch  InputPortMessageModes=m  OutputPortMessageModes=m,m  SwitchingCriterion=From attribute  Seed=9647085  SwitchAttributeName=trust
  Entity Output Switch8 : EntityOutputSwitch  InputPortMessageModes=m  OutputPortMessageModes=m,m  SwitchingCriterion=From attribute  Seed=9632160  SwitchAttributeName=extra_check
  Entity Output Switch9 : EntityOutputSwitch  InputPortMessageModes=m  OutputPortMessageModes=m,m  SwitchingCriterion=From attribute  Seed=9632160  SwitchAttributeName=extra_check
  Entity Queue2 : Queue  InputPortMessageModes=m  OutputPortMessageModes=m  Capacity=Inf
  Entity Queue3 : Queue  InputPortMessageModes=m  OutputPortMessageModes=m  Capacity=inf
  Entity Queue4 : Queue  InputPortMessageModes=m  OutputPortMessageModes=m  Capacity=inf
  Entity Replicator2 : EntityReplicator  InputPortMessageModes=m  OutputPortMessageModes=m,m
  Entity Replicator3 : EntityReplicator  InputPortMessageModes=m  OutputPortMessageModes=m,m
  Max1 : MinMax  Function=max  Inputs=2
  Tq{7..12} (6 alike) : Display
  Tw{7..12} (6 alike) : Display
  ρ{7..12} (6 alike) : Display
  Out1 : Outport
  Out2 : Outport  Port=2
  Out3 : Outport  Port=3
  Out4 : Outport  Port=4
  Out5 : Outport  Port=5
  Out6 : Outport  Port=6
  Out7 : Outport  Port=7
  Out8 : Outport  Port=8
  wires:
  In1/1 -> Entity Output Switch6/1
  Entity Queue2/1 -> Entity Output Switch7/1
  Entity Output Switch7/2 -> B9/1(In1)
  Entity Output Switch6/1 -> Entity Output Switch1/1
  Entity Output Switch6/2 -> Entity Queue2/1
  Entity Output Switch7/1 -> Entity Queue4/1
  Entity Output Switch1/1 -> Entity Queue3/1
  B7/1(Out2) -> Out2/1
  Entity Output Switch10/2 -> Out1/1
  B7/4(Out4) -> Tq8/1
  Entity Output Switch10/1 -> Entity Output Switch9/1
  B6/4(Out4) -> Tq7/1
  B7/5(Out5) -> Entity Input Switch9/1
  B8/4(Out4) -> Tq9/1
  B10/1(Out2) -> Out7/1
  Entity Output Switch9/1 -> Entity Input Switch10/1
  B6/3(Out3) -> ρ7/1
  B9/1(Out2) -> Out8/1
  D1/2(Out1) -> Tq10/1
  B7/3(Out3) -> ρ8/1
  Entity Replicator3/1 -> Entity Input Switch6/1
  B8/2(Out1) -> Tw9/1, Max1/2
  B8/1(Out2) -> Out5/1
  Entity Input Switch6/1 -> B7/1(In1)
  Entity Queue3/1 -> Entity Replicator3/1
  Entity Replicator2/1 -> Entity Input Switch6/2
  D1/4(Out4) -> Tw10/1
  Entity Replicator2/2 -> Entity Input Switch7/2
  Entity Input Switch7/1 -> B8/1(In1)
  D1/3(Out3) -> ρ10/1
  B6/1(Out2) -> Out4/1
  Entity Queue4/1 -> Entity Input Switch8/1
  B9/5(Out5) -> Entity Input Switch8/2
  B9/3(Out3) -> ρ11/1
  B6/2(Out1) -> Tw7/1
  D1/1(Out2) -> Out6/1
  Entity Replicator3/2 -> Entity Input Switch7/1
  B9/4(Out4) -> Tq11/1
  Entity Input Switch8/1 -> B10/1(In1)
  B10/2(Out1) -> [C2], Tw12/1
  B6/5(Out5) -> Entity Replicator2/1
  B10/3(Out3) -> ρ12/1
  Entity Output Switch8/2 -> Entity Input Switch11/2
  B9/2(Out1) -> Tw11/1
  Entity Input Switch11/1 -> D1/1(In1)
  B8/5(Out5) -> Entity Input Switch9/2
  D1/5(Out5) -> Entity Input Switch10/2
  Entity Output Switch9/2 -> Entity Input Switch11/1
  Entity Input Switch9/1 -> Entity Output Switch10/1
  Max1/1 -> ?
  B10/5(Out5) -> Entity Output Switch8/1
  B7/2(Out1) -> Max1/1, Tw8/1
  Entity Input Switch10/1 -> C1/1
  Entity Output Switch1/2 -> B6/1(In1)
  C1/1 -> Out3/1
  Entity Output Switch8/1 -> Entity Input Switch10/3
  B8/3(Out3) -> ρ9/1
  B10/4(Out4) -> Tq12/1
